simulink model "Rejz3"  (R2021a)
settings: Solver=VariableStepAuto  StartTime=0.0  StopTime=20.0  RelTol=1e-3
values from neighbouring files (symbols this model uses):
  C = [ 1 0 0 0 ]    [maj18.m]
  F = Phi - G*C*Phi    [maj18.m]
  G = Gt'    [maj18.m]
  Gamma = d_sys.b    [maj18.m]
  H = Gamma - G*C*Gamma    [maj18.m]
  K = acker(Phi, Gamma, [z1 z2 zcinf zcinf])    [maj18.m]
  Nu = Nxu(end)    [maj18.m]
  Nx = Nxu(1:4)    [maj18.m]
  Phi = d_sys.a    [maj18.m]
  Ts = 0.1    [maj18.m]
settings Model: Creator=Peti  LastModifiedBy=Peti

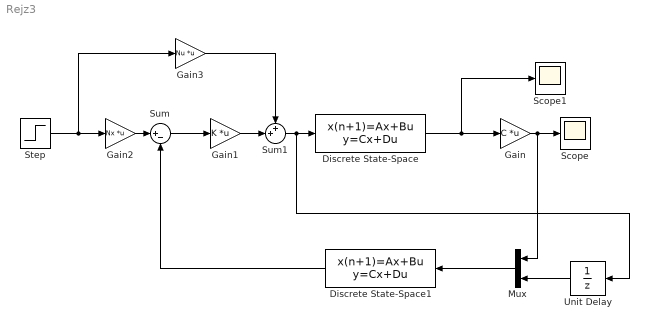
== system Rejz3 ==
  Discrete State-Space : DiscreteStateSpace  A=Phi  B=Gamma  C=eye(4)  D=zeros(4,1)  InitialCondition=[0 -0.05 0 0]  SampleTime=Ts
  Discrete State-Space1 : DiscreteStateSpace  A=F  B=[G H]  C=eye(4)  D=zeros(4,2)  InitialCondition=[0 -0.05 0 0]  SampleTime=Ts
  Gain : Gain  Gain=C  Multiplication=Matrix(K*u)
  Gain1 : Gain  Gain=K  Multiplication=Matrix(K*u)
  Gain2 : Gain  Gain=Nx  Multiplication=Matrix(K*u)
  Gain3 : Gain  Gain=Nu  Multiplication=Matrix(K*u)
  Mux : Mux  Inputs=2
  Scope : Scope
  Scope1 : Scope
  Step : Step  SampleTime=0
  Sum : Sum  Inputs=|+-
  Sum1 : Sum  Inputs=++|
  Unit Delay : UnitDelay  SampleTime=-1  HasFrameUpgradeWarning=on
  wires:
  Discrete State-Space/1 -> Scope1/1, Gain/1
  Gain/1 -> Mux/1, Scope/1
  Gain2/1 -> Sum/1
  Gain1/1 -> Sum1/2
  Sum1/1 -> Unit Delay/1, Discrete State-Space/1
  Gain3/1 -> Sum1/1
  Sum/1 -> Gain1/1
  Step/1 -> Gain3/1, Gain2/1
  Mux/1 -> Discrete State-Space1/1
  Unit Delay/1 -> Mux/2
  Discrete State-Space1/1 -> Sum/2
